simulink model "Extended_model_s"  (R2021b)
settings: Solver=VariableStepAuto  StartTime=0.0  StopTime=10.0  RelTol=1e-3
values from neighbouring files (symbols this model uses):
  Ask = [0 1 0 0 ... (first row only)    [H_inf_ctrl.m]    (also in H_inf_ctrl_11_2_p.m; H_inf_ctrl_11_3_heavy.m; H_inf_ctrl_11_3_light.m)
  Bsk = [0 0 0 0 ... (first row only)    [H_inf_ctrl.m]    (also in H_inf_ctrl_11_2_p.m; H_inf_ctrl_11_3_heavy.m; H_inf_ctrl_11_3_light.m)
  Csk = [0 1 0 0 ... (first row only)    [H_inf_ctrl.m]    (also in H_inf_ctrl_11_2_p.m; H_inf_ctrl_11_3_heavy.m; H_inf_ctrl_11_3_light.m)
  Dsk = zeros(2,4)    [H_inf_ctrl.m]    (also in H_inf_ctrl_11_2_p.m; H_inf_ctrl_11_3_heavy.m; H_inf_ctrl_11_3_light.m)
libraries: cstblocks x4
settings Model: LastModifiedBy=rivaa
settings OptimizationCC: BlockReduction=off  BooleanDataType=off
settings DebuggingCC: SaveWithParameterizedLinksMsg=none  UnderspecifiedInitializationDetection=Classic  MergeDetectMultiDrivingBlocksExec=none  SignalResolutionControl=TryResolveAllWithWarning
settings HardwareCC: TargetUnknown=on
settings ModelReferenceCC: PropagateSignalLabelsOutOfModel=off

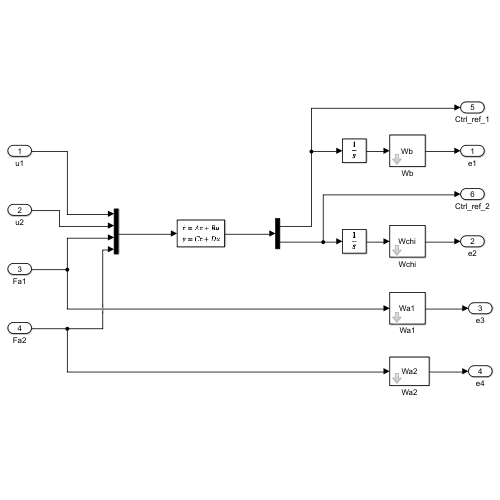
[thumbnail: Simulink's stored preview of the top-level diagram]
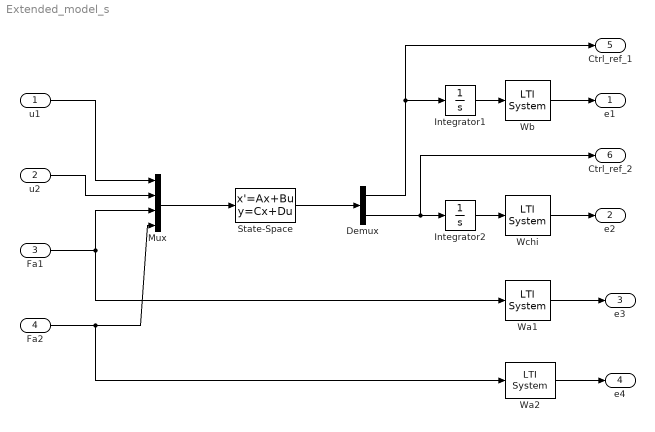
== system Extended_model_s ==
  u1 : Inport
  u2 : Inport  Port=2
  Fa1 : Inport  Port=3
  Fa2 : Inport  Port=4
  Demux : Demux  Outputs=2
  Integrator1 : Integrator
  Integrator2 : Integrator
  Mux : Mux
  State-Space : StateSpace  A=Ask  B=Bsk  C=Csk  D=Dsk  InitialCondition=0
  Wa1 : cstblocks/LTI System  sys=Wa1  IC=[]
  Wa2 : cstblocks/LTI System  sys=Wa2  IC=[]
  Wb : cstblocks/LTI System  sys=Wb  IC=[]
  Wchi : cstblocks/LTI System  sys=Wchi  IC=[]
  e1 : Outport
  e2 : Outport  Port=2
  e3 : Outport  Port=3
  e4 : Outport  Port=4
  Ctrl_ref_1 : Outport  Port=5
  Ctrl_ref_2 : Outport  Port=6
  wires:
  u1/1 -> Mux/1
  u2/1 -> Mux/2
  Fa1/1 -> Mux/3, Wa1/1
  Fa2/1 -> Mux/4, Wa2/1
  Wa1/1 -> e3/1
  Wa2/1 -> e4/1
  Mux/1 -> State-Space/1
  State-Space/1 -> Demux/1
  Demux/1 -> Ctrl_ref_1/1, Integrator1/1
  Demux/2 -> Ctrl_ref_2/1, Integrator2/1
  Wb/1 -> e1/1
  Wchi/1 -> e2/1
  Integrator1/1 -> Wb/1
  Integrator2/1 -> Wchi/1
